simulink model "get_started_simple_flow"  (R2023b)
settings: Solver=VariableStepAuto  StartTime=0.0  StopTime=10.0  RelTol=1e-3  AbsTol=1e-3
libraries: simulink x4
CloseFcn:
  | try,close(h1_ChokedFlowInGasOrifice),end
  | clear h1_ChokedFlowInGasOrifice
  | 
  | clear simlog_ChokedFlowInGasOrifice tout
Description:
  | Choked Flow in Gas Orifice
settings Model: Creator=The MathWorks, Inc.  LastModifiedBy=kroblet
settings SolverCC: AutoScaleAbsTol=off  AlgebraicLoopSolver=TrustRegion  MaxZcPerStep=1
settings DataIOCC: ReturnWorkspaceOutputs=off
settings DebuggingCC: UnconnectedInputMsg=warning  UnconnectedOutputMsg=warning  UnconnectedLineMsg=warning  PregeneratedLibrarySubsystemCodeDiagnostic=none  ArithmeticOperatorsInVariantConditions=warning
settings ModelReferenceCC: EnableRefExpFcnMdlSchedulingChecks=on
settings SFSimCC: SimUseLocalCustomCode=off  CustomCodeUndefinedFunction=UseInterfaceOnly
settings RTWCC: RTWUseLocalCustomCode=off  DLArmComputeVersion=19.05
settings CodeAppCC: StateflowObjectComments=on
settings GRTTargetCC: TargetLangStandard=C89/C90 (ANSI)
settings ConfigComp: CovMetricSettings=dsw  CovSaveCumulativeToWorkspaceVar=on  CovSaveSingleToWorkspaceVar=on  CovExternalEMLEnable=off
settings SimscapeCC: SimscapeLogType=all  SimscapeLogSimulationStatistics=on  SimscapeLogName=simlog_ChokedFlowInGasOrifice  SimscapeLogDataHistory=10000

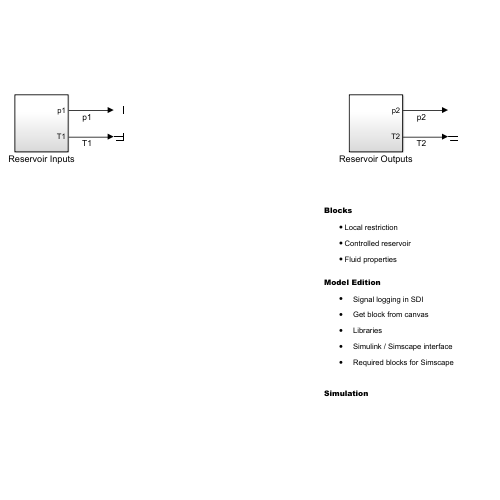
[thumbnail: Simulink's stored preview of the top-level diagram]
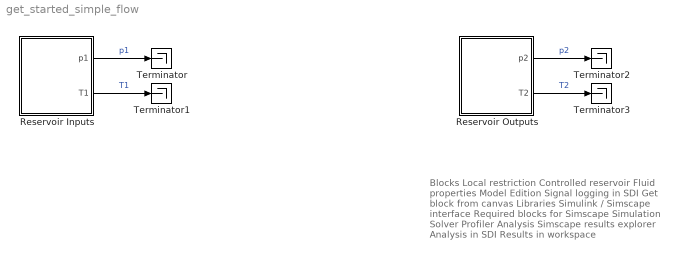
== system get_started_simple_flow ==
  note: Blocks
      | Local restriction
      | Controlled reservoir
      | Fluid properties
      | Model Edition
      | Signal logging in SDI
      | Get block from canvas
      | Libraries
      | Simulink / Simscape interface
      | Required blocks for Simscape
      | Simulation
      | Solver Profiler
      | Analysis
      | Simscape results explorer
      | Analysis in SDI
      | Results in workspace
  Reservoir Inputs : Subsystem
  Reservoir Outputs : Subsystem
  Terminator{,1..3} (4 alike) : Terminator
  wires:
  Reservoir Inputs/1(p1) -> Terminator/1  "p1"
  Reservoir Inputs/2(T1) -> Terminator1/1  "T1"
  Reservoir Outputs/2(T2) -> Terminator3/1  "T2"
  Reservoir Outputs/1(p2) -> Terminator2/1  "p2"

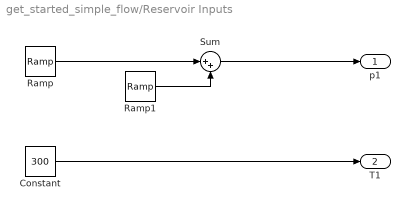
== system get_started_simple_flow/Reservoir Inputs ==
  Constant : Constant  Value=300
  Ramp : simulink/Sources/Ramp  slope=0.1  start=6  InitialOutput=0.5
  Ramp1 : simulink/Sources/Ramp  slope=-0.1  start=9  InitialOutput=0
  Sum : Sum  Inputs=|++
  p1 : Outport
  T1 : Outport  Port=2
  wires:
  Constant/1 -> T1/1
  Ramp1/1 -> Sum/2
  Ramp/1 -> Sum/1
  Sum/1 -> p1/1

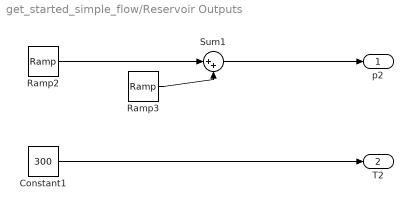
== system get_started_simple_flow/Reservoir Outputs ==
  Constant1 : Constant  Value=300
  Ramp2 : simulink/Sources/Ramp  slope=-0.075  start=1  InitialOutput=0.5
  Ramp3 : simulink/Sources/Ramp  slope=0.075  start=5  InitialOutput=0
  Sum1 : Sum  Inputs=|++
  p2 : Outport
  T2 : Outport  Port=2
  wires:
  Constant1/1 -> T2/1
  Sum1/1 -> p2/1
  Ramp2/1 -> Sum1/1
  Ramp3/1 -> Sum1/2
